simulink library "asbCubeSatDynamicsLib"  (R2021a)
settings: Solver=VariableStepAuto  StartTime=0.0  StopTime=10.0  RelTol=1e-3
undefined symbols (not defined in the file): initCond, vehicle
libraries: aerolibcubesatveh x3, sharedtransform x3
settings Model: Creator=The MathWorks, Inc.  LastModifiedBy=The MathWorks, Inc.
settings SolverCC: AlgebraicLoopSolver=TrustRegion
settings DataIOCC: ReturnWorkspaceOutputs=off
settings DebuggingCC: SFMachineParentedDataDiag=warning  ArithmeticOperatorsInVariantConditions=warning

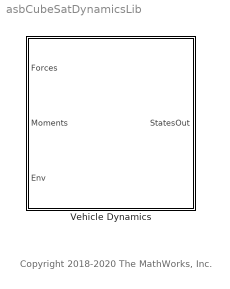
== system asbCubeSatDynamicsLib ==
  note: Copyright 2018-2020 The MathWorks, Inc.
  Vehicle Dynamics : Subsystem

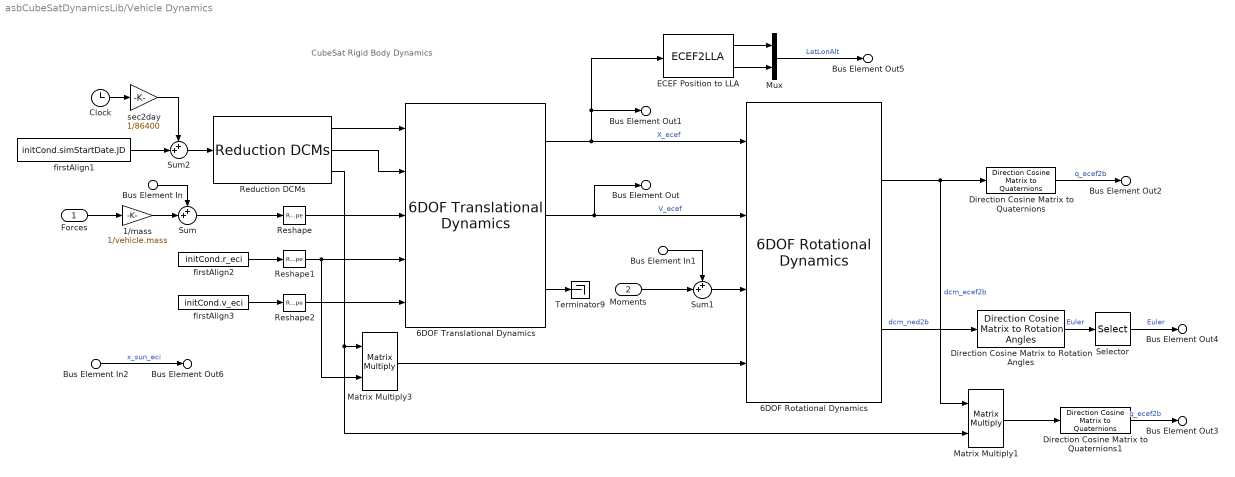
== system asbCubeSatDynamicsLib/Vehicle Dynamics ==
  note: CubeSat Rigid Body Dynamics
  Forces : Inport  RequirementInfo={} %GIDa_3bff085b_b60a_4e83_9a79_ee4d75de2c18
  Moments : Inport  RequirementInfo={} %GIDa_de23e7b3_b020_4a27_8ea7_dbdbe2a400f3  Port=2
  Bus Element In : Inport  Port=3  PortName=Env  Element=envAccel_ecef
  Bus Element In1 : Inport  Port=3  PortName=Env  Element=envTorques_body
  Bus Element In2 : Inport  Port=3  PortName=Env  Element=x_sun_eci
  1/mass : Gain  Gain=1/vehicle.mass
  6DOF Rotational Dynamics : aerolibcubesatveh/CubeSat Vehicle (Nadir Pointing)/6DOF Rotational Dynamics  euler0=initCond.euler  pqr0=initCond.pqr  inertia=vehicle.inertia
      settings: SourceProductBaseCode=AE
  6DOF Translational Dynamics : aerolibcubesatveh/CubeSat Vehicle (Nadir Pointing)/6DOF Translational Dynamics  SystemSampleTime=-1  VariantActivationTime=update diagram  Latency=0  AutoFrameSizeCalculation=off
      settings: SourceProductBaseCode=AE
  Clock : Clock
  Direction Cosine Matrix to Rotation Angles : sharedtransform/Direction Cosine Matrix to Rotation Angles  rotationOrder=ZYX  aMode=aMode  action=None  tolerance=eps(2)
      settings: SourceProductBaseCode=AE,PW,DR,MT,UV,VE
  Direction Cosine Matrix to Quaternions : sharedtransform/Direction Cosine Matrix  to Quaternions  RequirementInfo={} %GIDa_f6acb073_5fc2_4121_8cd8_59723b754a8d  aMode=aMode  action=None  tolerance=eps(2)
      settings: SourceProductBaseCode=AE,PW,DR,MT,UV,VE
  Direction Cosine Matrix to Quaternions1 : sharedtransform/Direction Cosine Matrix  to Quaternions  RequirementInfo={} %GIDa_ae7365ec_19bf_438b_9c86_285bc7c9a4ad  aMode=aMode  action=None  tolerance=eps(2)
      settings: SourceProductBaseCode=AE,PW,DR,MT,UV,VE
  ECEF Position to LLA : ECEF2LLA
  Matrix Multiply1 : Product  Multiplication=Matrix(*)
  Matrix Multiply3 : Product  Multiplication=Matrix(*)
  Mux : Mux  Inputs=2
  Reduction DCMs : aerolibcubesatveh/CubeSat Vehicle (Nadir Pointing)/Reduction DCMs
      settings: SourceProductBaseCode=AE
  Reshape : Reshape
  Reshape1 : Reshape
  Reshape2 : Reshape
  Selector : Selector  InputPortWidth=3  IndexOptions=Index vector (dialog)  Indices=[3 2 1]  OutputSizes=1
  Sum : Sum  RequirementInfo={} %GIDa_93ce11cd_3bb8_4d3a_a1de_f1041c0e8540  Inputs=++|
  Sum1 : Sum  RequirementInfo={} %GIDa_6da28457_7485_4e17_8924_3ed2b0e1d29f  Inputs=++|
  Sum2 : Sum  Inputs=++|
  Terminator9 : Terminator
  firstAlign1 : Constant  Value=initCond.simStartDate.JD  OutDataTypeStr=Inherit: Inherit via back propagation
  firstAlign2 : Constant  Value=initCond.r_eci  OutDataTypeStr=Inherit: Inherit via back propagation
  firstAlign3 : Constant  Value=initCond.v_eci  OutDataTypeStr=Inherit: Inherit via back propagation
  sec2day : Gain  Gain=1/86400
  Bus Element Out : Outport  VectorParamsAs1DForOutWhenUnconnected=off  PortName=StatesOut  Element=V_ecef
  Bus Element Out1 : Outport  VectorParamsAs1DForOutWhenUnconnected=off  PortName=StatesOut  Element=X_ecef
  Bus Element Out2 : Outport  VectorParamsAs1DForOutWhenUnconnected=off  PortName=StatesOut  Element=q_ecef2b
  Bus Element Out3 : Outport  VectorParamsAs1DForOutWhenUnconnected=off  PortName=StatesOut  Element=q_eci2b
  Bus Element Out4 : Outport  VectorParamsAs1DForOutWhenUnconnected=off  PortName=StatesOut  Element=Euler
  Bus Element Out5 : Outport  VectorParamsAs1DForOutWhenUnconnected=off  PortName=StatesOut  Element=LatLonAlt
  Bus Element Out6 : Outport  VectorParamsAs1DForOutWhenUnconnected=off  PortName=StatesOut  Element=x_sun_eci
  wires:
  Direction Cosine Matrix to Quaternions1/1 -> Bus Element Out3/1  "q_ecef2b"
  Matrix Multiply1/1 -> Direction Cosine Matrix to Quaternions1/1
  ECEF Position to LLA/1 -> Mux/1
  ECEF Position to LLA/2 -> Mux/2
  6DOF Rotational Dynamics/1 -> Direction Cosine Matrix to Quaternions/1, Matrix Multiply1/1  "dcm_ecef2b"
  Reshape2/1 -> 6DOF Translational Dynamics/5
  firstAlign3/1 -> Reshape2/1
  Reshape1/1 -> 6DOF Translational Dynamics/4, Matrix Multiply3/2
  Reshape/1 -> 6DOF Translational Dynamics/3
  firstAlign2/1 -> Reshape1/1
  Matrix Multiply3/1 -> 6DOF Rotational Dynamics/4
  Reduction DCMs/3 -> Matrix Multiply3/1, Matrix Multiply1/2
  Sum/1 -> Reshape/1
  Forces/1 -> 1/mass/1
  6DOF Translational Dynamics/3 -> Terminator9/1
  Reduction DCMs/2 -> 6DOF Translational Dynamics/2
  Reduction DCMs/1 -> 6DOF Translational Dynamics/1
  Sum1/1 -> 6DOF Rotational Dynamics/3
  Moments/1 -> Sum1/2
  Bus Element In1/1 -> Sum1/1
  Bus Element In2/1 -> Bus Element Out6/1  "x_sun_eci"
  6DOF Translational Dynamics/1 -> ECEF Position to LLA/1, Bus Element Out1/1, 6DOF Rotational Dynamics/1  "X_ecef"
  6DOF Rotational Dynamics/2 -> Direction Cosine Matrix to Rotation Angles/1  "dcm_ned2b"
  Direction Cosine Matrix to Rotation Angles/1 -> Selector/1  "Euler"
  Direction Cosine Matrix to Quaternions/1 -> Bus Element Out2/1  "q_ecef2b"
  6DOF Translational Dynamics/2 -> Bus Element Out/1, 6DOF Rotational Dynamics/2  "V_ecef"
  Mux/1 -> Bus Element Out5/1  "LatLonAlt"
  Clock/1 -> sec2day/1
  Sum2/1 -> Reduction DCMs/1
  firstAlign1/1 -> Sum2/2
  sec2day/1 -> Sum2/1
  Selector/1 -> Bus Element Out4/1  "Euler"
  1/mass/1 -> Sum/2
  Bus Element In/1 -> Sum/1
